simulink model "cs_recharge_model"  (R2026a)
settings: Solver=ode45  StopTime=1000
settings Model: Creator=keiyasoda  LastModifiedBy=keiyasoda

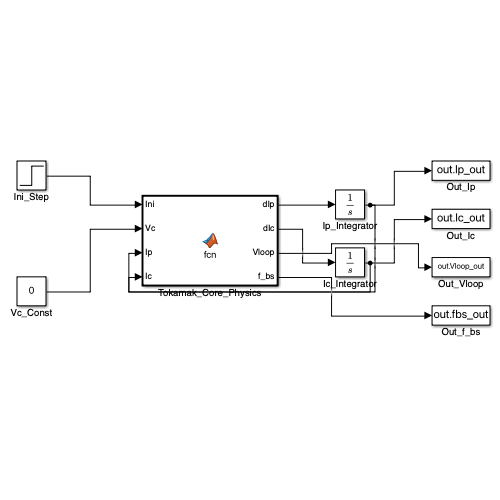
[thumbnail: Simulink's stored preview of the top-level diagram]
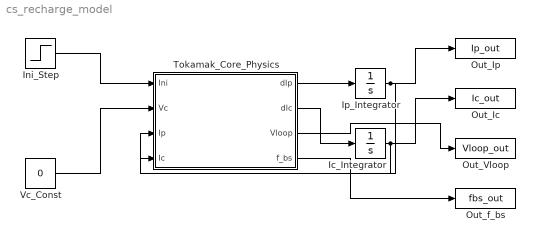
== system cs_recharge_model ==
  Ic_Integrator : Integrator  InitialCondition=3.0e4
  Ini_Step : Step  Time=200  InitialValue=1.75e6  FinalValue=9.5e6  SampleTime=0
  Ip_Integrator : Integrator  InitialCondition=7.0e6
  Out_Ic : ToWorkspace  VariableName=Ic_out  SaveFormat=Timeseries  SampleTime=-1
  Out_Ip : ToWorkspace  VariableName=Ip_out  SaveFormat=Timeseries  SampleTime=-1
  Out_Vloop : ToWorkspace  VariableName=Vloop_out  SaveFormat=Timeseries  SampleTime=-1
  Out_f_bs : ToWorkspace  VariableName=fbs_out  SaveFormat=Timeseries  SampleTime=-1
  Tokamak_Core_Physics : MATLAB Function  TreatAsAtomicUnit=on
  Vc_Const : Constant  Value=0
  wires:
  Ini_Step/1 -> Tokamak_Core_Physics/1(Ini)
  Vc_Const/1 -> Tokamak_Core_Physics/2(Vc)
  Tokamak_Core_Physics/1(dIp) -> Ip_Integrator/1
  Tokamak_Core_Physics/2(dIc) -> Ic_Integrator/1
  Ip_Integrator/1 -> Tokamak_Core_Physics/3(Ip), Out_Ip/1
  Ic_Integrator/1 -> Tokamak_Core_Physics/4(Ic), Out_Ic/1
  Tokamak_Core_Physics/3(Vloop) -> Out_Vloop/1
  Tokamak_Core_Physics/4(f_bs) -> Out_f_bs/1

== matlab function cs_recharge_model/Tokamak_Core_Physics ==
  data: Ini input; dIp output; Vc input; Ip input; Ic input; dIc output; Vloop output; f_bs output
function [dIp, dIc, Vloop, f_bs] = fcn(Ini, Vc, Ip, Ic)
    % FAST Tokamak Device Parameters
    Lp = 5.0e-6;   % Plasma self-inductance (H)
    Lc = 0.5;      % Central Solenoid self-inductance (H)
    M  = 1.2e-3;   % Mutual inductance (H)
    Rp = 1.0e-8;   % Plasma resistance (Spitzer-like at high Te)
    Rc = 0.0;      % Superconducting HTS magnet resistance
    Ip_nominal = 7.0e6; 

    % State Derivatives Matrix Solution
    denom = (Lp * Lc) - (M^2);
    dIp = (Lc * Rp * (Ini - Ip) - M * (Vc - Rc * Ic)) / denom;
    dIc = (-M * Rp * (Ini - Ip) + Lp * (Vc - Rc * Ic)) / denom;

    % Diagnostic Outputs
    Vloop = Rp * (Ip - Ini);
    % Calculate Bootstrap Fraction based on standard DT profile metrics
    f_bs = (Ini * 0.4) / Ip_nominal;
end
